simulink model "MIL"  (R2023a)
settings: Solver=VariableStepAuto  StartTime=0.0  StopTime=2  RelTol=1e-3
libraries: SignalEditorBlockLib x1
settings Model: Creator=eslam  LastModifiedBy=eslam

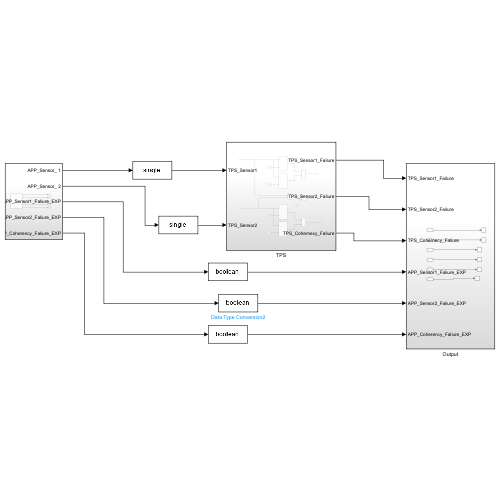
[thumbnail: Simulink's stored preview of the top-level diagram]
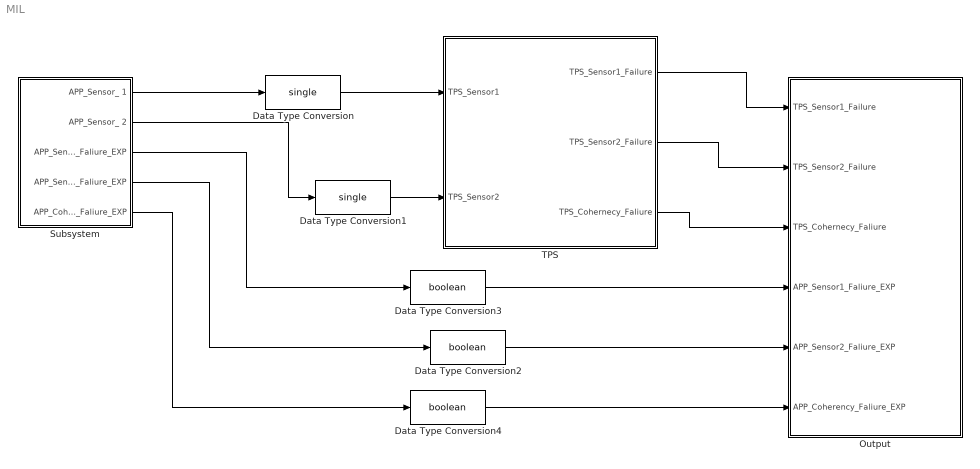
== system MIL ==
  Data Type Conversion : DataTypeConversion  OutDataTypeStr=single  SaturateOnIntegerOverflow=off  RndMeth=Floor
  Data Type Conversion1 : DataTypeConversion  OutDataTypeStr=single  SaturateOnIntegerOverflow=off  RndMeth=Floor
  Data Type Conversion2 : DataTypeConversion  OutDataTypeStr=boolean  SaturateOnIntegerOverflow=off  RndMeth=Floor
  Data Type Conversion3 : DataTypeConversion  OutDataTypeStr=boolean  SaturateOnIntegerOverflow=off  RndMeth=Floor
  Data Type Conversion4 : DataTypeConversion  OutDataTypeStr=boolean  SaturateOnIntegerOverflow=off  RndMeth=Floor
  Output : Subsystem
  Subsystem : Subsystem
  TPS : Subsystem
  wires:
  Subsystem/1(APP_Sensor_ 1) -> Data Type Conversion/1
  TPS/1(TPS_Sensor1_Failure) -> Output/1(TPS_Sensor1_Failure)
  TPS/2(TPS_Sensor2_Failure) -> Output/2(TPS_Sensor2_Failure)
  TPS/3(TPS_Cohernecy_Faliure) -> Output/3(TPS_Cohernecy_Faliure)
  Subsystem/2(APP_Sensor_ 2) -> Data Type Conversion1/1
  Subsystem/3(APP_Sensor1_Faliure_EXP) -> Data Type Conversion3/1
  Subsystem/4(APP_Sensor2_Faliure_EXP) -> Data Type Conversion2/1
  Subsystem/5(APP_Coherency_Faliure_EXP) -> Data Type Conversion4/1
  Data Type Conversion/1 -> TPS/1(TPS_Sensor1)
  Data Type Conversion1/1 -> TPS/2(TPS_Sensor2)
  Data Type Conversion3/1 -> Output/4(APP_Sensor1_Faliure_EXP)
  Data Type Conversion2/1 -> Output/5(APP_Sensor2_Faliure_EXP)
  Data Type Conversion4/1 -> Output/6(APP_Coherency_Faliure_EXP)

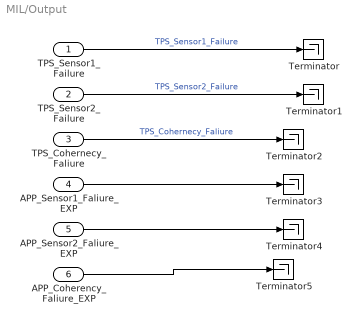
== system MIL/Output ==
  TPS_Sensor1_Failure : Inport
  TPS_Sensor2_Failure : Inport  Port=2
  TPS_Cohernecy_Faliure : Inport  Port=3
  APP_Sensor1_Faliure_EXP : Inport  Port=4
  APP_Sensor2_Faliure_EXP : Inport  Port=5
  APP_Coherency_Faliure_EXP : Inport  Port=6
  Terminator{,1..5} (6 alike) : Terminator
  wires:
  TPS_Sensor1_Failure/1 -> Terminator/1  "TPS_Sensor1_Failure"
  TPS_Cohernecy_Faliure/1 -> Terminator2/1  "TPS_Cohernecy_Faliure"
  APP_Sensor1_Faliure_EXP/1 -> Terminator3/1
  APP_Sensor2_Faliure_EXP/1 -> Terminator4/1
  APP_Coherency_Faliure_EXP/1 -> Terminator5/1
  TPS_Sensor2_Failure/1 -> Terminator1/1  "TPS_Sensor2_Failure"

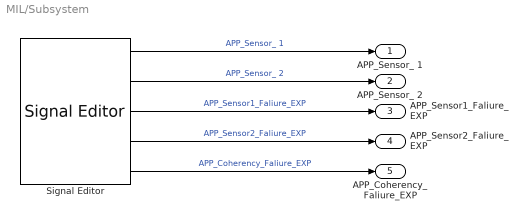
== system MIL/Subsystem ==
  Signal Editor : SignalEditorBlockLib/Signal Editor  FileName=C:\Users\eslam\Downloads\TechnicalPart\MILTest.mat  ActiveScenario=Sheet1  ActiveSignal=TPS_vSensor_1  IsBus=off  OutputBusObjectStr=Bus: BusObject  SampleTime=0  Interpolate=off  ZeroCross=off  OutputAfterFinalValue=Setting to zero  Unit=inherit  PreserveSignalName=on  ApplySigPropsToAllScenarios=on
  APP_Sensor_ 1 : Outport
  APP_Sensor_ 2 : Outport  Port=2
  APP_Sensor1_Faliure_EXP : Outport  Port=3
  APP_Sensor2_Faliure_EXP : Outport  Port=4
  APP_Coherency_Faliure_EXP : Outport  Port=5
  wires:
  Signal Editor/1 -> APP_Sensor_ 1/1  "APP_Sensor_ 1"
  Signal Editor/3 -> APP_Sensor1_Faliure_EXP/1  "APP_Sensor1_Faliure_EXP"
  Signal Editor/5 -> APP_Coherency_Faliure_EXP/1  "APP_Coherency_Faliure_EXP"
  Signal Editor/4 -> APP_Sensor2_Faliure_EXP/1  "APP_Sensor2_Faliure_EXP"
  Signal Editor/2 -> APP_Sensor_ 2/1  "APP_Sensor_ 2"

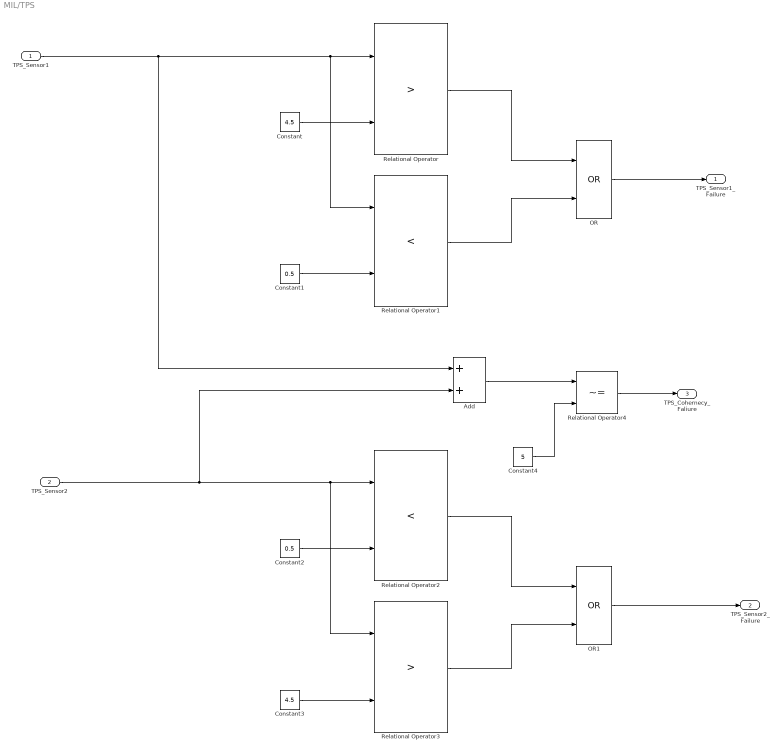
== system MIL/TPS ==
  TPS_Sensor1 : Inport  OutDataTypeStr=single
  TPS_Sensor2 : Inport  Port=2  OutDataTypeStr=single
  Add : Sum
  Constant : Constant  Value=4.5
  Constant1 : Constant  Value=0.5
  Constant2 : Constant  Value=0.5
  Constant3 : Constant  Value=4.5
  Constant4 : Constant  Value=5
  OR : Logic  Operator=OR  AllPortsSameDT=off  OutDataTypeStr=boolean
  OR1 : Logic  Operator=OR  AllPortsSameDT=off  OutDataTypeStr=boolean
  Relational Operator : RelationalOperator  Operator=>  OutDataTypeStr=boolean  RndMeth=Simplest  InputSameDT=off
  Relational Operator1 : RelationalOperator  Operator=<  OutDataTypeStr=boolean  RndMeth=Simplest  InputSameDT=off
  Relational Operator2 : RelationalOperator  Operator=<  OutDataTypeStr=boolean  RndMeth=Simplest  InputSameDT=off
  Relational Operator3 : RelationalOperator  Operator=>  OutDataTypeStr=boolean  RndMeth=Simplest  InputSameDT=off
  Relational Operator4 : RelationalOperator  Operator=~=  OutDataTypeStr=boolean  RndMeth=Simplest  InputSameDT=off
  TPS_Sensor1_Failure : Outport  OutDataTypeStr=boolean
  TPS_Sensor2_Failure : Outport  Port=2  OutDataTypeStr=boolean
  TPS_Cohernecy_Faliure : Outport  Port=3  OutDataTypeStr=boolean
  wires:
  Constant/1 -> Relational Operator/2
  OR/1 -> TPS_Sensor1_Failure/1
  Relational Operator/1 -> OR/1
  Constant1/1 -> Relational Operator1/2
  Relational Operator1/1 -> OR/2
  TPS_Sensor1/1 -> Add/1, Relational Operator1/1, Relational Operator/1
  Constant3/1 -> Relational Operator3/2
  Constant2/1 -> Relational Operator2/2
  Relational Operator2/1 -> OR1/1
  TPS_Sensor2/1 -> Add/2, Relational Operator3/1, Relational Operator2/1
  Relational Operator3/1 -> OR1/2
  OR1/1 -> TPS_Sensor2_Failure/1
  Add/1 -> Relational Operator4/1
  Constant4/1 -> Relational Operator4/2
  Relational Operator4/1 -> TPS_Cohernecy_Faliure/1
